simulink model "Caso9ControleRele"  (R2015a)
settings: Solver=ode45  StartTime=0.0  StopTime=10  RelTol=1e-3
settings Model: Creator=user  LastModifiedBy=user
settings SolverCC: ZeroCrossControl=DisableAll

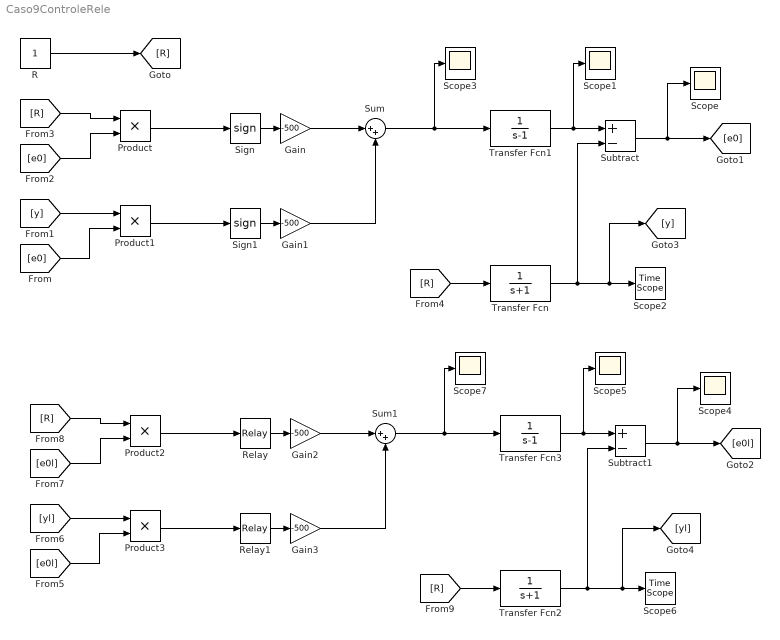
== system Caso9ControleRele ==
  Gain{,1..3} (4 alike) : Gain  Gain=-500
  Product{,1..3} (4 alike) : Product
  R : Constant
  Relay : Relay  OnSwitchValue=0.05  OffSwitchValue=-0.05  OffOutputValue=-1
  Relay1 : Relay  OnSwitchValue=0.05  OffSwitchValue=-0.05  OffOutputValue=-1
  Scope{,1,3..5,7} (6 alike) : Scope
      Scope settings: YMin=-1.73472e-18  YMax=0.02
      Scope1 settings: YMin=0.1  YMax=1
      Scope3 settings: YMin=-525  YMax=-475  SaveName=ScopeData3
      Scope4 settings: YMin=-1.73472e-18  YMax=0.02  SaveName=ScopeData2
      Scope5 settings: YMin=5.55112e-17  YMax=1.1  SaveName=ScopeData4
      Scope7 settings: YMin=-525  YMax=-475  SaveName=ScopeData6
  Scope2 : TimeScope
  Scope6 : TimeScope
  Sign : Signum
  Sign1 : Signum
  Subtract : Sum  Inputs=+-
  Subtract1 : Sum  Inputs=+-
  Sum : Sum  Inputs=|++
  Sum1 : Sum  Inputs=|++
  Transfer Fcn : TransferFcn  Denominator=[1 1]
  Transfer Fcn1 : TransferFcn  Denominator=[1 -1]
  Transfer Fcn2 : TransferFcn  Denominator=[1 1]
  Transfer Fcn3 : TransferFcn  Denominator=[1 -1]
  wires:
  Sum/1 -> Scope3/1, Transfer Fcn1/1
  Sign/1 -> Gain/1
  Sign1/1 -> Gain1/1
  Gain1/1 -> Sum/2
  Gain/1 -> Sum/1
  Product/1 -> Sign/1
  Product1/1 -> Sign1/1
  [e0] -> Product1/2
  [y] -> Product1/1
  [e0] -> Product/2
  [R] -> Product/1
  [R] -> Transfer Fcn/1
  Transfer Fcn1/1 -> Scope1/1, Subtract/1
  Transfer Fcn/1 -> Subtract/2, [y], Scope2/1
  Subtract/1 -> Scope/1, [e0]
  R/1 -> [R]
  Sum1/1 -> Scope7/1, Transfer Fcn3/1
  Relay/1 -> Gain2/1
  Relay1/1 -> Gain3/1
  Gain3/1 -> Sum1/2
  Gain2/1 -> Sum1/1
  Product2/1 -> Relay/1
  Product3/1 -> Relay1/1
  [e0l] -> Product3/2
  [yl] -> Product3/1
  [e0l] -> Product2/2
  [R] -> Product2/1
  [R] -> Transfer Fcn2/1
  Transfer Fcn3/1 -> Scope5/1, Subtract1/1
  Transfer Fcn2/1 -> Subtract1/2, [yl], Scope6/1
  Subtract1/1 -> Scope4/1, [e0l]
